simulink model "SSC_LQR"  (R2024b)
settings: Solver=VariableStepAuto  StartTime=0.0  StopTime=10.0  RelTol=1e-3
undefined symbols (not defined in the file or in its folder): drv, rpm2rads, ssc_LQR
settings Model: Creator=llp  LastModifiedBy=llp

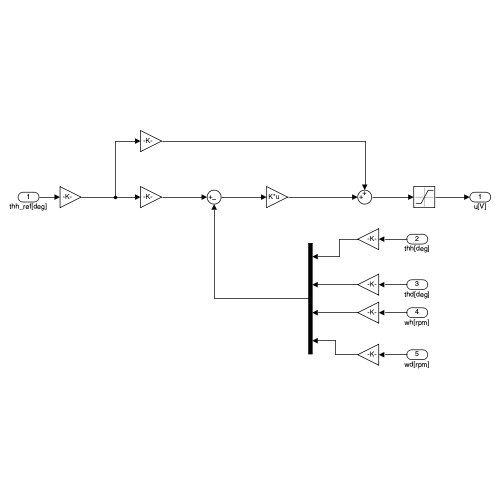
[thumbnail: Simulink's stored preview of the top-level diagram]
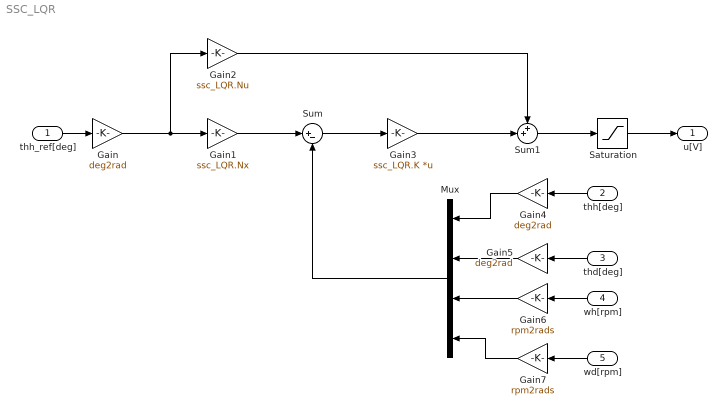
== system SSC_LQR ==
  thh_ref[deg] : Inport
  thh[deg] : Inport  Port=2
  thd[deg] : Inport  Port=3
  wh[rpm] : Inport  Port=4
  wd[rpm] : Inport  Port=5
  Gain : Gain  Gain=deg2rad
  Gain1 : Gain  Gain=ssc_LQR.Nx
  Gain2 : Gain  Gain=ssc_LQR.Nu
  Gain3 : Gain  Gain=ssc_LQR.K  Multiplication=Matrix(K*u)
  Gain4 : Gain  Gain=deg2rad
  Gain5 : Gain  Gain=deg2rad
  Gain6 : Gain  Gain=rpm2rads
  Gain7 : Gain  Gain=rpm2rads
  Mux : Mux
  Saturation : Saturate  UpperLimit=drv.outmax  LowerLimit=-drv.outmax
  Sum : Sum  Inputs=|+-
  Sum1 : Sum  Inputs=++|
  u[V] : Outport
  wires:
  Gain7/1 -> Mux/4
  Gain2/1 -> Sum1/1
  Gain4/1 -> Mux/1
  Gain/1 -> Gain2/1, Gain1/1
  Gain3/1 -> Sum1/2
  Saturation/1 -> u[V]/1
  thh_ref[deg]/1 -> Gain/1
  Mux/1 -> Sum/2
  wd[rpm]/1 -> Gain7/1
  Gain5/1 -> Mux/2
  thh[deg]/1 -> Gain4/1
  Sum/1 -> Gain3/1
  thd[deg]/1 -> Gain5/1
  Gain1/1 -> Sum/1
  wh[rpm]/1 -> Gain6/1
  Gain6/1 -> Mux/3
  Sum1/1 -> Saturation/1
